simulink model "State_machine_test"  (R2017b)
settings: Solver=VariableStepAuto  StartTime=0.0  StopTime=10.0  RelTol=1e-3
settings Model: Creator=Kalana  LastModifiedBy=Kalana

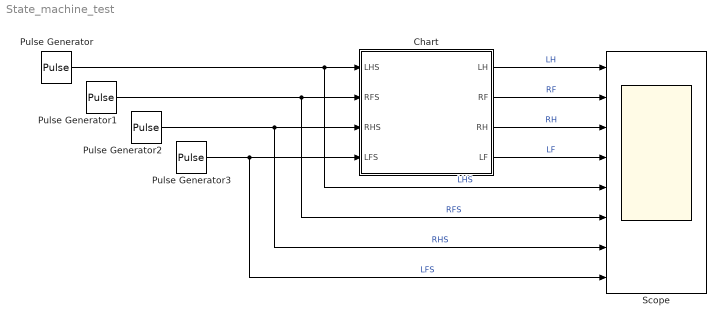
== system State_machine_test ==
  Chart : Stateflow chart  TreatAsAtomicUnit=on
  Pulse Generator : DiscretePulseGenerator  PulseType=Time based  PulseWidth=50
  Pulse Generator1 : DiscretePulseGenerator  PulseType=Time based  PulseWidth=50
  Pulse Generator2 : DiscretePulseGenerator  PulseType=Time based  PulseWidth=50  PhaseDelay=1
  Pulse Generator3 : DiscretePulseGenerator  PulseType=Time based  PulseWidth=50  PhaseDelay=1
  Scope : Scope  NumInputPorts=8
  wires:
  Chart/2(RF) -> Scope/2  "RF"
  Chart/4(LF) -> Scope/4  "LF"
  Chart/3(RH) -> Scope/3  "RH"
  Chart/1(LH) -> Scope/1  "LH"
  Pulse Generator/1 -> Scope/5, Chart/1(LHS)  "LHS"
  Pulse Generator1/1 -> Scope/6, Chart/2(RFS)  "RFS"
  Pulse Generator2/1 -> Scope/7, Chart/3(RHS)  "RHS"
  Pulse Generator3/1 -> Scope/8, Chart/4(LFS)  "LFS"

== stateflow chart State_machine_test/Chart ==
  state LF_RH_swing
    entry: LF = 0
    RF = 1
    RH = 0
    LH = 1
  state Intermediate
    entry: LF = LF
    RF = RF
    RH = RH
    LH = LH
  state RF_LH_swing
    entry: LF = 1
    RF = 0
    RH = 1
    LH = 0
  LF_RH_swing -> Intermediate : [LFS + RHS]
  Intermediate -> RF_LH_swing [order 1] : [LFS*RHS]
  (default) -> LF_RH_swing
  Intermediate -> LF_RH_swing [order 2] : [RFS*LHS]
  RF_LH_swing -> Intermediate : [RFS+LHS]
  data: LHS input; RFS input; RHS input; LH output; RF output; RH output; LF output; LFS input
